simulink model "mpc_uncon_Kailin"  (R2019b)
settings: Solver=VariableStepAuto  StartTime=0.0  StopTime=time_end  RelTol=1e-3
values from neighbouring files (symbols this model uses):
  A = [1 0 0 0 0 0 0 1 0 0 0 0 ... (36 elements, 6x6)]    [quadcopter_data_unc.mat]
  B = [0 0.0254156742081 0.00196363636364 0 0.508313484163 0.0392727272727 0.0254156742081 0 -0.00196363636364 0.508313484163 0 -0.0392727272727 ... (24 elements, 6x4)]    [quadcopter_data_unc.mat]
  C = [1 0 0 0 1 0 0 0 1 0 0 0 ... (18 elements, 3x6)]    [quadcopter_data_unc.mat]
  F = [F; C*A^i]    [cal_mpc_matrix.m]    (also in quadcopter_data_unc.mat = [1 0 0 1 0 0 1 0 0 1 0 0 ... (180 elements, 30x6)])
  G = [G; C * innter_mat * B]    [cal_mpc_matrix.m]    (also in quadcopter_data_unc.mat = [0 0.0254156742081 0.00196363636364 0 0.101662696833 0.00785)
  h_01 = 10.17    [script_mpc_uncon.m]
  h_02 = 10.53    [script_mpc_uncon.m]
  K = zero_filter * K_full    [cal_mpc_matrix.m]    (also in quadcopter_data_unc.mat = [2.75363895013e-19 0.0115834228675 -2.53706105467e-19 -0.011)
  ue = [ue1; ue2]    [script_mpc_uncon.m]
  xe = [xe1; xe2]    [script_mpc_uncon.m]
  xe2 = 25.53    [script_mpc_uncon.m]
settings Model: Creator=NicSch02  LastModifiedBy=tongk

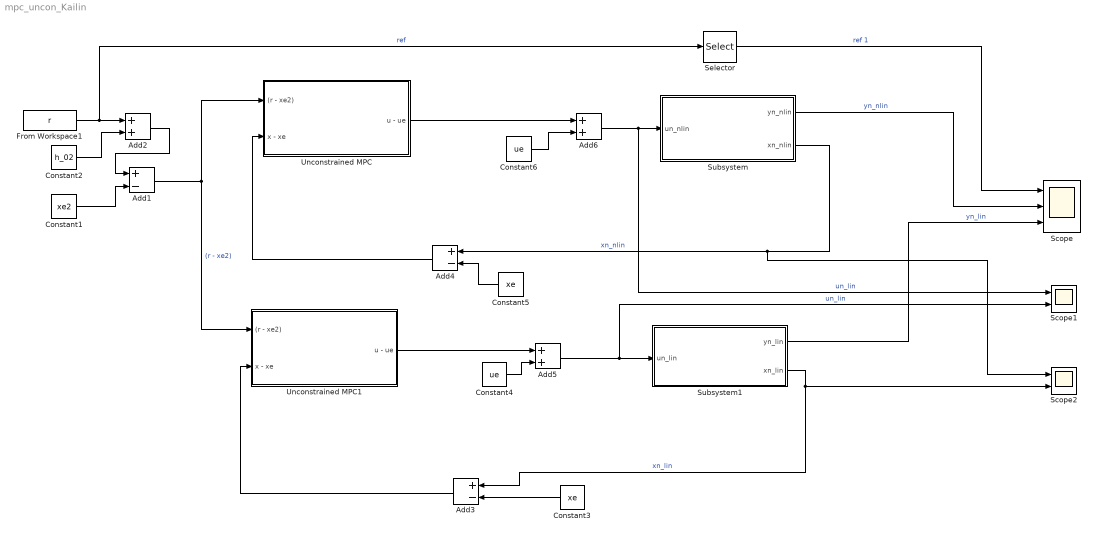
== system mpc_uncon_Kailin ==
  Add1 : Sum  Inputs=+-
  Add2 : Sum
  Add3 : Sum  Inputs=+-
  Add4 : Sum  Inputs=+-
  Add5 : Sum
  Add6 : Sum
  Constant1 : Constant  Value=xe2
  Constant2 : Constant  Value=h_02
  Constant3 : Constant  Value=xe
  Constant4 : Constant  Value=ue
  Constant5 : Constant  Value=xe
  Constant6 : Constant  Value=ue
  From Workspace1 : FromWorkspace  VariableName=r  SampleTime=0
  Scope : Scope  NumInputPorts=3
  Scope1 : Scope  NumInputPorts=2
  Scope2 : Scope  NumInputPorts=2
  Selector : Selector  InputPortWidth=Np  IndexOptions=Index vector (dialog)  Indices=[1]  OutputSizes=1
  Subsystem : Subsystem
  Subsystem1 : Subsystem
  Unconstrained MPC : Subsystem
  Unconstrained MPC1 : Subsystem
  wires:
  Subsystem/1(yn_nlin) -> Scope/2  "yn_nlin"
  Add5/1 -> Scope1/2, Subsystem1/1(un_lin)  "un_lin"
  Subsystem/2(xn_nlin) -> Scope2/1, Add4/1  "xn_nlin"
  Subsystem1/2(xn_lin) -> Add3/1, Scope2/2  "xn_lin"
  Selector/1 -> Scope/1  "ref 1"
  Add2/1 -> Add1/1
  From Workspace1/1 -> Selector/1, Add2/1  "ref"
  Constant2/1 -> Add2/2
  Subsystem1/1(yn_lin) -> Scope/3  "yn_lin"
  Add1/1 -> Unconstrained MPC1/1((r - xe2)), Unconstrained MPC/1((r - xe2))  "(r - xe2)"
  Constant1/1 -> Add1/2
  Constant3/1 -> Add3/2
  Constant4/1 -> Add5/2
  Constant5/1 -> Add4/2
  Constant6/1 -> Add6/2
  Add6/1 -> Scope1/1, Subsystem/1(un_nlin)  "un_lin"
  Add4/1 -> Unconstrained MPC/2(x - xe)
  Unconstrained MPC/1(u - ue) -> Add6/1
  Unconstrained MPC1/1(u - ue) -> Add5/1
  Add3/1 -> Unconstrained MPC1/2(x - xe)

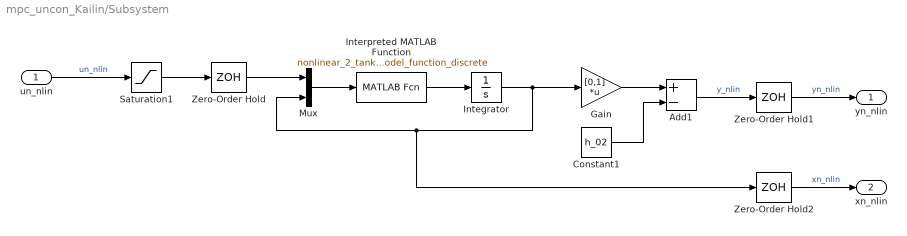
== system mpc_uncon_Kailin/Subsystem ==
  un_nlin : Inport
  Add1 : Sum  Inputs=+-
  Constant1 : Constant  Value=h_02
  Gain : Gain  Gain=[0,1]  Multiplication=Matrix(K*u)
  Integrator : Integrator  InitialCondition=[h_01;h_02]
  Interpreted MATLAB Function : MATLABFcn  MATLABFcn=nonlinear_2_tank_model_function_discrete
  Mux : Mux  Inputs=2
  Saturation1 : Saturate  UpperLimit=5  LowerLimit=0
  Zero-Order Hold : ZeroOrderHold  SampleTime=0.5
  Zero-Order Hold1 : ZeroOrderHold  SampleTime=0.5
  Zero-Order Hold2 : ZeroOrderHold  SampleTime=0.5
  yn_nlin : Outport
  xn_nlin : Outport  Port=2
  wires:
  Integrator/1 -> Zero-Order Hold2/1, Mux/2, Gain/1
  Constant1/1 -> Add1/2
  Interpreted MATLAB Function/1 -> Integrator/1
  Gain/1 -> Add1/1
  Mux/1 -> Interpreted MATLAB Function/1
  un_nlin/1 -> Saturation1/1  "un_nlin"
  Zero-Order Hold/1 -> Mux/1
  Add1/1 -> Zero-Order Hold1/1  "y_nlin"
  Zero-Order Hold1/1 -> yn_nlin/1  "yn_nlin"
  Saturation1/1 -> Zero-Order Hold/1
  Zero-Order Hold2/1 -> xn_nlin/1  "xn_nlin"

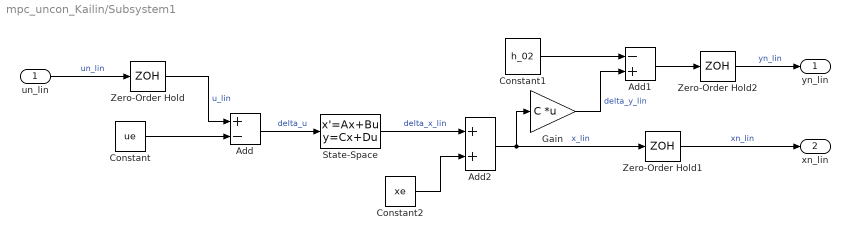
== system mpc_uncon_Kailin/Subsystem1 ==
  un_lin : Inport
  Add : Sum  Inputs=+-
  Add1 : Sum  Inputs=-+
  Add2 : Sum
  Constant : Constant  Value=ue
  Constant1 : Constant  Value=h_02
  Constant2 : Constant  Value=xe
  Gain : Gain  Gain=C  Multiplication=Matrix(K*u)
  State-Space : StateSpace  A=A  B=B  C=[[1,0];[0,1]]  D=[[0,0];[0,0]]  InitialCondition=[h_01;h_02] - xe
  Zero-Order Hold : ZeroOrderHold  SampleTime=-1
  Zero-Order Hold1 : ZeroOrderHold  SampleTime=-1
  Zero-Order Hold2 : ZeroOrderHold  SampleTime=-1
  yn_lin : Outport
  xn_lin : Outport  Port=2
  wires:
  Constant/1 -> Add/2
  Add/1 -> State-Space/1  "delta_u"
  Constant2/1 -> Add2/2
  State-Space/1 -> Add2/1  "delta_x_lin"
  un_lin/1 -> Zero-Order Hold/1  "un_lin"
  Zero-Order Hold/1 -> Add/1  "u_lin"
  Add2/1 -> Zero-Order Hold1/1, Gain/1  "x_lin"
  Zero-Order Hold1/1 -> xn_lin/1  "xn_lin"
  Zero-Order Hold2/1 -> yn_lin/1  "yn_lin"
  Add1/1 -> Zero-Order Hold2/1
  Constant1/1 -> Add1/1
  Gain/1 -> Add1/2  "delta_y_lin"

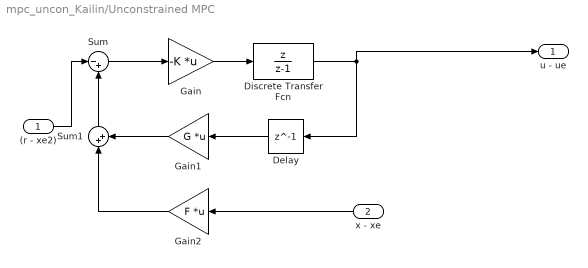
== system mpc_uncon_Kailin/Unconstrained MPC ==
  (r - xe2) : Inport
  x - xe : Inport  Port=2
  Delay : Delay  DelayLength=1
  Discrete Transfer Fcn : DiscreteTransferFcn  Numerator=[1 0]  Denominator=[1 -1]  SampleTime=0.5
  Gain : Gain  Gain=-K  Multiplication=Matrix(K*u)
  Gain1 : Gain  Gain=G  Multiplication=Matrix(K*u)
  Gain2 : Gain  Gain=F  Multiplication=Matrix(K*u)
  Sum : Sum  Inputs=|-+
  Sum1 : Sum  Inputs=|++
  u - ue : Outport
  wires:
  Gain1/1 -> Sum1/2
  Sum/1 -> Gain/1
  (r - xe2)/1 -> Sum/1
  x - xe/1 -> Gain2/1
  Discrete Transfer Fcn/1 -> u - ue/1, Delay/1
  Delay/1 -> Gain1/1
  Gain/1 -> Discrete Transfer Fcn/1
  Sum1/1 -> Sum/2
  Gain2/1 -> Sum1/1

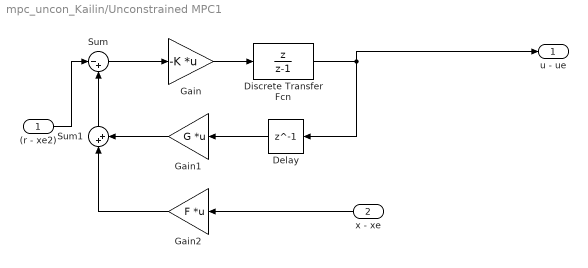
== system mpc_uncon_Kailin/Unconstrained MPC1 ==
  (r - xe2) : Inport
  x - xe : Inport  Port=2
  Delay : Delay  DelayLength=1
  Discrete Transfer Fcn : DiscreteTransferFcn  Numerator=[1 0]  Denominator=[1 -1]  SampleTime=0.5
  Gain : Gain  Gain=-K  Multiplication=Matrix(K*u)
  Gain1 : Gain  Gain=G  Multiplication=Matrix(K*u)
  Gain2 : Gain  Gain=F  Multiplication=Matrix(K*u)
  Sum : Sum  Inputs=|-+
  Sum1 : Sum  Inputs=|++
  u - ue : Outport
  wires:
  Gain1/1 -> Sum1/2
  Sum/1 -> Gain/1
  (r - xe2)/1 -> Sum/1
  x - xe/1 -> Gain2/1
  Discrete Transfer Fcn/1 -> u - ue/1, Delay/1
  Delay/1 -> Gain1/1
  Gain/1 -> Discrete Transfer Fcn/1
  Sum1/1 -> Sum/2
  Gain2/1 -> Sum1/1
